simulink model "LQG_tracker_simulink"  (R2025b)
settings: Solver=VariableStepAuto  StartTime=0.0  StopTime=10.0  RelTol=1e-3
values from neighbouring files (symbols this model uses):
  A = [ 0, 1, 0, 0 ... (first row only)    [Controller_LQR.m]    (also in H_inf_controller.m = zeros(4,4); Hinf.m = zeros(4,4); Hinf_tuner.m = zeros(4,4); LQG_controller.m = zeros(4,4))
  Ac_ctrl = [A - B*Kx - Kf*C, -B*Ki ... (first row only)    [LQG_controller.m]
  B = [0 ... (first row only)    [Controller_LQR.m]    (also in H_inf_controller.m = (dx_p - dx_m) / (2*h); Hinf.m = (dx_p - dx_m) / (2*h); Hinf_tuner.m = (dx_p - dx_m)/(2*h); LQG_controller.m = (dx_p - dx_m) / (2*h))
  Bc_ctrl = [zeros(4,1), Kf ... (first row only)    [LQG_controller.m]
  C = [1 0 0 0]    [Controller_LQR.m]    (also in H_inf_controller.m; Hinf.m; Hinf_tuner.m; LQG_controller.m)
  Cc_ctrl = [-Kx, -Ki]    [LQG_controller.m]
  D = 0    [Controller_LQR.m]    (also in H_inf_controller.m; Hinf.m; Hinf_tuner.m; LQG_controller.m)
  Dc_ctrl = [zeros(1,1), zeros(1,1)]    [LQG_controller.m]
settings Model: Creator=Administrator  LastModifiedBy=Administrator

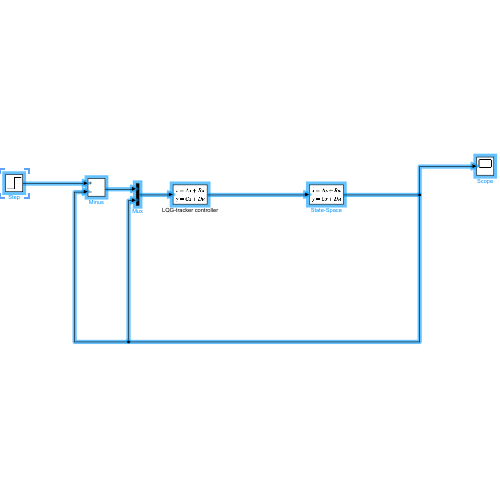
[thumbnail: Simulink's stored preview of the top-level diagram]
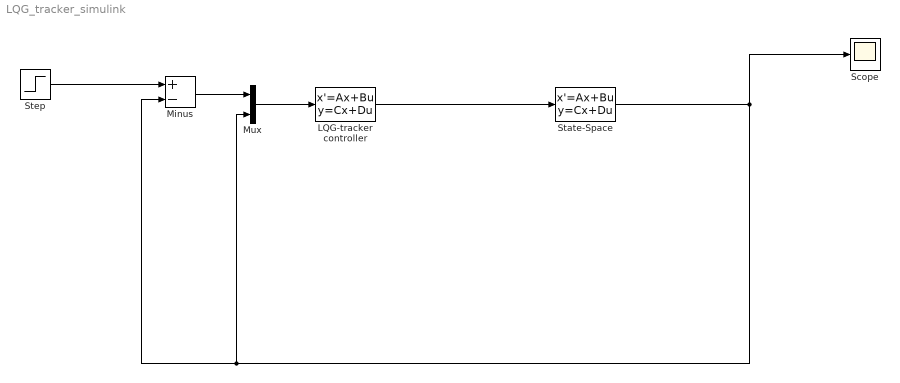
== system LQG_tracker_simulink ==
  LQG-tracker controller : StateSpace  A=Ac_ctrl  B=Bc_ctrl  C=Cc_ctrl  D=Dc_ctrl  InitialCondition=0
  Minus : Sum  Inputs=+-
  Mux : Mux  Inputs=2
  Scope : Scope
      settings: ActiveDisplayYMinimum=-0.1264885247503322  ActiveDisplayYMaximum=1.13839672275299
  State-Space : StateSpace  A=A  B=B  C=C  D=D  InitialCondition=0
  Step : Step  SampleTime=0
  wires:
  Step/1 -> Minus/1
  State-Space/1 -> Scope/1, Mux/2, Minus/2
  Minus/1 -> Mux/1
  Mux/1 -> LQG-tracker controller/1
  LQG-tracker controller/1 -> State-Space/1
